simulink library "lineFollowingApproach1"  (R2018b)
settings: Solver=VariableStepAuto  StartTime=0.0  StopTime=10.0  RelTol=1e-3
settings Model: Creator=anna  LastModifiedBy=anna

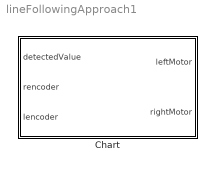
== system lineFollowingApproach1 ==
  Chart : Stateflow chart  TreatAsAtomicUnit=on

== stateflow chart lineFollowingApproach1/Chart ==
  state otherColor
  state blackColor
    entry:
    rightMotor = 40;
    leftMotor=40;
  state waiting
    entry:
    rightMotor =0 ;
    leftMotor=0;
    counter=40;
  state checkRight
    leftMotor = 30;
    rightMotor = -30;
  state go_to_beginning
    rightMotor = 30;
    leftMotor = -30;
  state checkLeft1
    rightMotor = 30;
    leftMotor = -30;
  state go_to_beginning1
    rightMotor = -30;
    leftMotor = 20;
  (junction 59) -> blackColor
  (junction 58) -> (junction 59)
  (default) -> otherColor : {remember=0;}
  otherColor -> blackColor [order 1] : [detectedValue==1]
  checkRight -> blackColor [order 1] : [detectedValue==1]{remember=0;}
  blackColor -> waiting : [detectedValue~=1]
  otherColor -> waiting [order 2] : [detectedValue~=1]
  waiting -> (junction 76) [order 2] : [remember==1]{lencoderStarting = lencoder;rencoderStarting = rencoder;}
  waiting -> checkRight [order 1] : [remember==0]{lencoderStarting = lencoder;rencoderStarting = rencoder;}
  (junction 76) -> checkLeft1
  checkRight -> go_to_beginning [order 3] : [abs(lencoder-lencoderStarting)>counter]
  go_to_beginning -> checkLeft1 : [lencoder<=lencoderStarting]{counter=counter+10;}
  go_to_beginning1 -> checkRight : [rencoder<=rencoderStarting]{counter=counter+10;}
  checkRight -> checkRight [order 2] : [abs(lencoder-lencoderStarting)<=counter && detectedValue~=1]
  checkLeft1 -> (junction 58) [order 1] : [detectedValue==1]{remember=1;}
  checkLeft1 -> checkLeft1 [order 2] : [abs(rencoder-rencoderStarting)<=counter && detectedValue~=1]
  checkLeft1 -> go_to_beginning1 [order 3] : [abs(rencoder-rencoderStarting)>counter]
  data: detectedValue input; leftMotor output; rightMotor output; rencoder input; rencoderStarting local; lencoderStarting local; lencoder input; counter local; remember local
